simulink model "DriverInLoopGamingEngine"  (R2022b)
settings: Solver=ode3  StartTime=0.0  StopTime=inf  FixedStep=1e-3  RelTol=1e-3
StartFcn:
  | tg.load('DriverInLoopSpeedgoat');
  | tg.start;
StopFcn:
  | tg.stop;
model workspace (MAT data in the model file):
  DLCXref = [0 7.023 7.5 18 33 33.5 45 50 60]
  DLCYref = [0 0 -4.5 -4.25 -3.75 1.5 1.25 0 0]
  Downshift_Speeds = [9.5625  23.0625  36.5625  47.8125  59.0625  68.90625  78.75; 12.9375  26.4375  39.9375  51.1875  62.4375  72.84375  83.25; 16.3125  29.8125  43.3125  54.5625  65.8125  76.78125  87.75; 19.6875  33.1875  46.6875  57.9375  69.1875  80.71875  92.25]
  EngRevLim = 7000
  Pedal_Positions = [0.1 0.4 0.5 0.9]
  Upshift_Speeds = [12.9375  26.4375  39.9375  51.1875  62.4375  72.84375  83.25; 16.3125  29.8125  43.3125  54.5625  65.8125  76.78125  87.75; 19.6875  33.1875  46.6875  57.9375  69.1875  80.71875  92.25; 33  52.5  77.25  100.5  138.75  161.875  185]
  VEH.Mass = 1181
  VEH.StaticNormalFrontLoad.FR = 264.666666667
  VEH.StaticNormalFrontLoad.FL = 264.666666667
  VEH.StaticNormalRearLoad.RR = 322
  VEH.StaticNormalRearLoad.RL = 322
  VEH.WheelBase = 3.075
  VEH.FrontAxlePositionfromCG = 1.515
  VEH.RearAxlePositionfromCG = 1.504
  VEH.HeightCG = 0.134
  VEH.FrontalArea = 2.11
  VEH.DragCoefficient = 0.33
  VEH.NumberOfWheelsPerAxle = 2
  VEH.PitchMomentInertia = 1922.66666667
  VEH.RollMomentInertia = 432.333333333
  VEH.YawMomentInertia = 2066
  VEH.SteeringRatio = 18
  VEH.TrackWidth = 1.922
  VEH.SprungMass = 1096.72266667
  VEH.InitialLongPosition = -26
  VEH.InitialLatPosition = 76
  VEH.InitialVertPosition = 0
  VEH.InitialRollAngle = 0
  VEH.InitialPitchAngle = 0
  VEH.InitialYawAngle = -0.698131700798
  VEH.InitialLongVel = 0
  VEH.InitialLatVel = 0
  VEH.InitialVertVel = 0
  VEH.InitialRollRate = 0
  VEH.InitialPitchRate = 0
  VEH.InitialYawRate = 0
libraries: slrealtimeutilitieslib x3, slrealtimeiplib x3, sim3dlib x2, sim3dautolib x1, vrlib x1, simulink x1
settings Model: Creator=ashankar  LastModifiedBy=RASLab-Distributed
settings SolverCC: AlgebraicLoopSolver=TrustRegion  AutoInsertRateTranBlk=on  InsertRTBMode=Never (minimum delay)  DecoupledContinuousIntegration=on
settings DebuggingCC: UnconnectedInputMsg=warning  UnconnectedOutputMsg=warning  UnconnectedLineMsg=warning  SFMachineParentedDataDiag=warning  ArithmeticOperatorsInVariantConditions=warning
settings ModelReferenceCC: EnableRefExpFcnMdlSchedulingChecks=on
settings SFSimCC: SimUseLocalCustomCode=off  CustomCodeUndefinedFunction=UseInterfaceOnly
settings RTWCC: RTWUseLocalCustomCode=off  DLArmComputeVersion=19.05

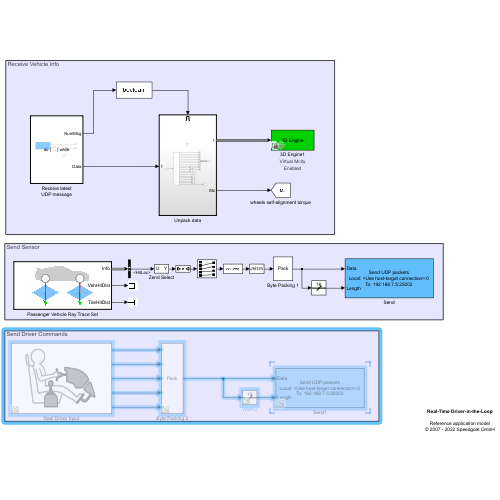
[thumbnail: Simulink's stored preview of the top-level diagram]
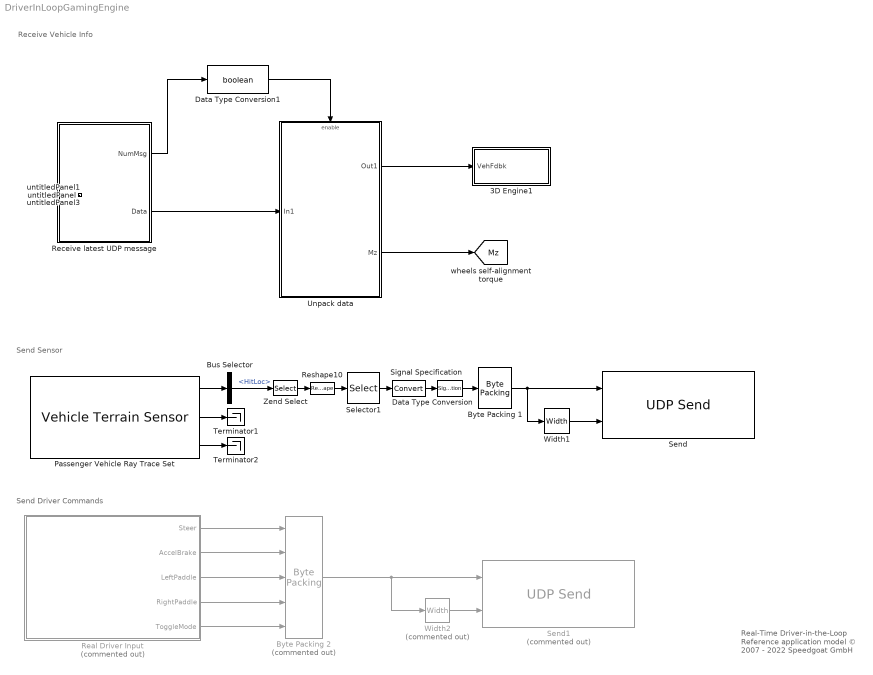
== system DriverInLoopGamingEngine ==
  note: Send Sensor
  note: Receive Vehicle Info
  note: Send Driver Commands
  note: Real-Time Driver-in-the-Loop
      |
      | Reference application model
      | © 2007 - 2022 Speedgoat GmbH
  3D Engine1 : Subsystem  Variant=on  VariantControlMode=label  LabelModeActiveChoice=1  mask(3D Engine){engine3D=Enabled, SceneDesc=Virtual Mcity, dt3D=0.02, defaultPos=Recommended for scene, X_o=-26.0, Y_o=76.0, Z_o=0.0, phi_o=0, theta_o=0, psi_o=-40*pi/180}
      mask prompts: engine3D "3D Engine"; SceneDesc "Scene:"; dt3D "Engine frame rate, dt3D [s]:"; X_o "Initial longitudinal position, X_o [m]:"; Y_o "Initial lateral position, Y_o [m]:"; Z_o "Initial vertical position, Z_o [m]:"; phi_o "Initial roll angle, phi_o [rad]:"; theta_o "Initial pitch angle, theta_o [rad]:"; psi_o "Initial yaw angle, psi_o [rad]:"
      mask help: This subsystem contains the interface blocks which permit the display of the vehicle in the 3D virtual environment. Enable it to view the simulation progress, disable it to inhibit the display.
      mask init:
      | switch get_param(gcb,'engine3D')
      |     case 'Disabled'
      |         set_param(gcb,'OverrideUsingVariant','0')
      |         try
      |             set_param([bdroot '/Environment/Ground Feedback'],'OverrideUsingVariant','0')
      |         catch
      |             disp('Warning: No ground feedback sensor not set')
      |         end
      |     case 'Enabled'
      |         set_param(gcb,'OverrideUsingVariant','1')
      |         try
      |             set_param([bdroot '/Environment/Ground Feedback'],'OverrideUsingVariant','1')
      |         catch
      |             disp('Warning: No ground feedback sensor not set')
      |         end
      |     otherwise
      |         set_param(gcb,'OverrideUsingVariant','0')
      | end
      settings: AttributesFormatString=|
      | %<SceneDesc>
      | %<engine3D>
      mask Help: eval('vdynblkshelp(''vdynblks3dengine'')');
      mask TypeOptions engine3D: Enabled | Disabled
      mask Callback engine3D:
      | switch get_param(gcb,'engine3D')
      |     case 'Disabled'
      |         set_param(gcb,'OverrideUsingVariant','0')
      |     case 'Enabled'
      |        set_param(gcb,'OverrideUsingVariant','1')
      |     otherwise
      |        set_param(gcb,'OverrideUsingVariant','0')
      | end
      mask TypeOptions SceneDesc: 3D Engine/Simulation 3D Scene Configuration/SceneDesc
      mask Callback SceneDesc:
      | defaultStatus = get_param(gcb,'defaultPos');
      | if strcmp(defaultStatus,'Recommended for scene')
      | sceneType = get_param(gcb,'SceneDesc');
      | switch sceneType
      |     case 'Straight road'
      |         set_param(gcb,'X_o', '-118')
      |         set_param(gcb,'Y_o', '3.125')
      |         set_param(gcb,'Z_o', '0')
      |         set_param(gcb,'phi_o', '0')
      |         set_param(gcb,'theta_o', '0')
      |         set_param(gcb,'psi_o', '0')
      |     case 'Curved road'
      |         set_param(gcb,'X_o', '0.2')
      |         set_param(gcb,'Y_o', '-1605.0')
      |         set_param(gcb,'Z_o', '0')
      |         set_param(gcb,'phi_o', '0')
      |         set_param(gcb,'theta_o', '0')
      |         set_param(gcb,'psi_o', '-156*pi/180')
      |     case 'Parking lot'
      |         set_param(gcb,'X_o', '-104.0')
      |         set_param(gcb,'Y_o', '-9.7')
      |         set_param(gcb,'Z_o', '0')
      |         set_param(gcb,'phi_o', '0')
      |         set_param(gcb,'theta_o', '0')
      |         set_param(gcb,'psi_o', '0')
      |     case 'Double lane change'
      |         set_param(gcb,'X_o', '0')
      |         set_param(gcb,'Y_o', '3.125')
      |         set_param(gcb,'Z_o', '0')
      |         set_param(gcb,'phi_o', '0')
      |         set_param(gcb,'theta_o', '0')
      |         set_param(gcb,'psi_o', '0')
      |     case 'Open surface'
      |         set_param(gcb,'X_o', '0')
      |         set_param(gcb,'Y_o', '0')
      |         set_param(gcb,'Z_o', '0')
      |         set_param(gcb,'phi_o', '0')
      |         set_param(gcb,'theta_o', '0')
      |         set_param(gcb,'psi_o', '0')
      |     case 'US highway'
      |         set_param(gcb,'X_o', '3592.00')
      |         set_param(gcb,'Y_o', '2617.00')
      |         set_param(gcb,'Z_o', '-1.0')
      |         set_param(gcb,'phi_o', '0')
      |         set_param(gcb,'theta_o', '0')
      |         set_param(gcb,'psi_o', '0')
      |     case 'US city block'
      |         set_param(gcb,'X_o', '-125.19')
      |         set_param(gcb,'Y_o', '1.65')
      |         set_param(gcb,'Z_o', '-0.04')
      |         set_param(gcb,'phi_o', '0')
      |         set_param(gcb,'theta_o', '0')
      |         set_param(gcb,'psi_o', '0')
      |     case 'Large parking lot'
      |         set_param(gcb,'X_o', '45.0')
      |         set_param(gcb,'Y_o', '54.7')
      |         set_param(gcb,'Z_o', '0.0')
      |         set_param(gcb,'phi_o', '0')
      |         set_param(gcb,'theta_o', '0')
      |         set_param(gcb,'psi_o', '-pi/2')
      |     case 'Virtual Mcity'
      |         set_param(gcb,'X_o', '-26.0')
      |         set_param(gcb,'Y_o', '76.0')
      |         set_param(gcb,'Z_o', '0.0')
      |         set_param(gcb,'phi_o', '0')
      |         set_param(gcb,'theta_o', '0')
      |         set_param(gcb,'psi_o', '-40*pi/180')
      |     otherwise
      |         set_param(gcb,'X_o', '0')
      |         set_param(gcb,'Y_o', '0')
      |         set_param(gcb,'Z_o', '0')
      |         set_param(gcb,'phi_o', '0')
      |         set_param(gcb,'theta_o', '0')
      |         set_param(gcb,'psi_o', '0')
      | end
      | end
      mask TypeOptions defaultPos: Recommended for scene | User-specified
      mask DialogControl engineConfig Prompt: 3D Engine Settings
      mask DialogControl posSetup Prompt: Initial vehicle position
      mask DialogControl posSetupDesc Prompt: To use these initial vehicle positions, first Apply the initial values and then click Update the model workspaces with the initial values.
      mask DialogControl setModelPos Prompt: Update model workspaces with initial values
      mask DialogControl setModelPos Callback:
      | if strcmp(get_param(bdroot(gcb),'SimulationStatus'),'stopped')
      |     sceneType = get_param(gcb,'SceneDesc');
      |     rootModel = bdroot(gcb);
      |     ws = get_param(rootModel, 'modelworkspace');
      |     VEH = getVariable(ws,'VEH');
      |     ParamList={'X_o',[1,1],{};'Y_o',[1,1],{};'Z_o',[1,1],{};'phi_o',[1,1],{'gte',-pi/2;'lte',pi/2};'theta_o',[1,1],{'gte',-pi/2;'lte',pi/2};'psi_o',[1,1],{'gte',-2*pi;'lte',2*pi}};
      |     paramStruct = autoblkscheckparams(gcb, '3D Engine',ParamList);
      |     VEH.InitialLongPosition = paramStruct.X_o;
      |     VEH.InitialLatPosition = paramStruct.Y_o;
      |     VEH.InitialVertPosition = paramStruct.Z_o;
      |     VEH.InitialRollAngle = paramStruct.phi_o;
      |     VEH.InitialPitchAngle = paramStruct.theta_o;
      |     VEH.InitialYawAngle = paramStruct.psi_o;
      |     assignin(ws,'VEH',VEH);
      |     modelList = {'PassVeh14DOF','PassVeh7DOF'};
      |     for idx =1:length(modelList)
      | %         try
      |             load_system(modelList{idx});
      |             ws = get_param(modelList{idx}, 'modelworkspace');
      |             assignin(ws,'VEH',VEH);
      |             save_system(modelList{idx});
      |             close_system(modelList{idx});
      | %         catch
      | %             disp(['Cannot find ' modelList{idx}])
      | %         end
      |     end
      | end
      mask Display: disp('3D Engine')
  Bus Selector : BusSelector  OutputSignals=HitLoc
  Byte Packing 1 : slrealtimeutilitieslib/Byte Packing  MaskPackedDataType=uint8  MaskUnpackedDataTypes={['single']}  MaskAlignment=1
  Byte Packing 2 : slrealtimeutilitieslib/Byte Packing  Commented=on  MaskPackedDataType=uint8  MaskUnpackedDataTypes={'double','double','boolean','boolean','boolean'}  MaskAlignment=1
  Data Type Conversion : DataTypeConversion  SaturateOnIntegerOverflow=off  RndMeth=Floor
  Data Type Conversion1 : DataTypeConversion  OutDataTypeStr=boolean  SaturateOnIntegerOverflow=off  RndMeth=Floor
  Passenger Vehicle Ray Trace Set : sim3dlib/Vehicle Terrain Sensor  Priority=1  ActorTag=SimulinkVehicle1  VehExtEn=Constant  TireRadiiExt=Constant  VehCntrLngthVal=0  TireRadiiVal=0  VehRayLngth=10  LfRayLngth=20  RfRayLngth=20  LrRayLngth=20  RrRayLngth=20  VehRayOffset=0  LfRayOffset=-1  RfRayOffset=-1  LrRayOffset=-1  RrRayOffset=-1  VehEn=on  LfEn=on  RfEn=on  LrEn=on  RrEn=on  DbgEn=off  Ts=-1  aMode=aMode
  Real Driver Input : Subsystem  Commented=on
      mask Display: image('LongitudinalDriver.png'); % Use "Edit Image" on toolstrip to change.
  Receive latest UDP message : Subsystem  TreatAsAtomicUnit=on
  Reshape10 : Reshape  OutputDimensionality=Row vector (2-D)
  Selector1 : Selector  InputPortWidth=5  IndexOptions=Index vector (dialog)  Indices=[2:5]  OutputSizes=1
  Send : slrealtimeiplib/UDP Send  useHostTargetConn=on  toAddress=target_ip  toPort=25002  sampleTime=-1  enableMessage=off  ipAddress=172.16.19.29  localPort=-1
  Send1 : slrealtimeiplib/UDP Send  Commented=on  useHostTargetConn=on  toAddress=target_ip  toPort=25003  sampleTime=-1  enableMessage=off  ipAddress=172.16.19.29  localPort=-1
  Signal Specification : SignalSpecification  Unit=m
  Terminator1 : Terminator
  Terminator2 : Terminator
  Unpack data : Subsystem
  Width1 : Width
  Width2 : Width  Commented=on
  Zend Select : Selector  NumberOfDimensions=2  InputPortWidth=3  IndexOptions=Select all,Index vector (dialog)  Indices=[1 3],3  OutputSizes=1,1
  untitledPanel : Subsystem  Tag=HiddenForWebPanel  IsWebBlockPanel=on
  untitledPanel1 : Subsystem  Tag=HiddenForWebPanel  IsWebBlockPanel=on
  untitledPanel3 : Subsystem  Tag=HiddenForWebPanel  IsWebBlockPanel=on
  tag scope: Mz=global
  wires:
  Reshape10/1 -> Selector1/1
  Bus Selector/1 -> Zend Select/1  "<HitLoc>"
  Zend Select/1 -> Reshape10/1
  Passenger Vehicle Ray Trace Set/3 -> Terminator2/1
  Passenger Vehicle Ray Trace Set/1 -> Bus Selector/1
  Width1/1 -> Send/2
  Passenger Vehicle Ray Trace Set/2 -> Terminator1/1
  Byte Packing 1/1 -> Width1/1, Send/1
  Width2/1 -> Send1/2
  Byte Packing 2/1 -> Width2/1, Send1/1
  Real Driver Input/2(AccelBrake) -> Byte Packing 2/2
  Real Driver Input/3(LeftPaddle) -> Byte Packing 2/3
  Real Driver Input/1(Steer) -> Byte Packing 2/1
  Real Driver Input/4(RightPaddle) -> Byte Packing 2/4
  Selector1/1 -> Data Type Conversion/1
  Data Type Conversion/1 -> Signal Specification/1
  Signal Specification/1 -> Byte Packing 1/1
  Data Type Conversion1/1 -> Unpack data/Enable
  Receive latest UDP message/2(Data) -> Unpack data/1(In1)
  Receive latest UDP message/1(NumMsg) -> Data Type Conversion1/1
  Real Driver Input/5(ToggleMode) -> Byte Packing 2/5
  Unpack data/2(Mz) -> [Mz]
  Unpack data/1(Out1) -> 3D Engine1/1(VehFdbk)

== system DriverInLoopGamingEngine/3D Engine1 ==
  note: 1) Add Subsystem or Model blocks as valid variant choices.
      | 2) You cannot connect blocks at this level. At simulation, connectivity is automatically
      | determined, based on the active variant and port name matching.
  VehFdbk : Inport
  3D Engine : Subsystem  VariantControl=1
  3D Engine Disabled : Subsystem  VariantControl=0

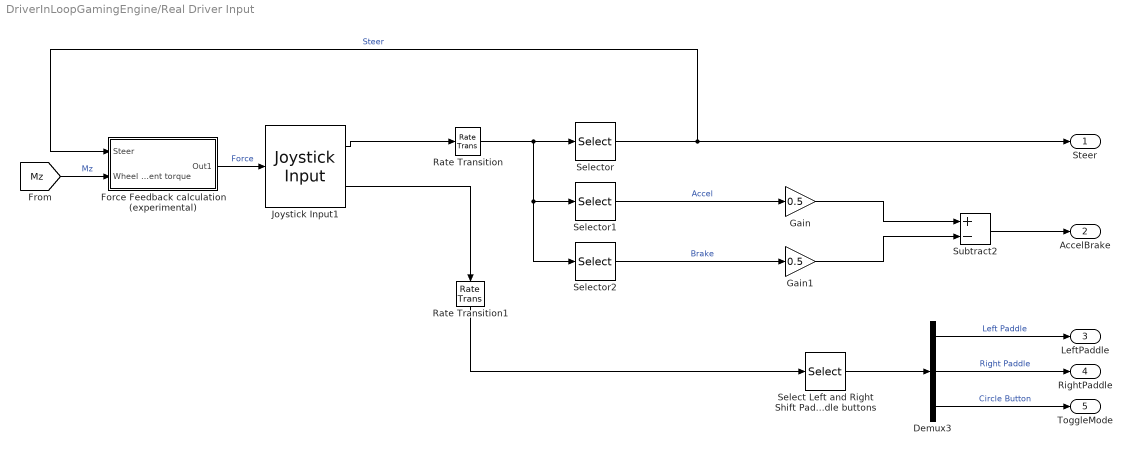
== system DriverInLoopGamingEngine/Real Driver Input ==
  Demux3 : Demux  Outputs=3
  Force Feedback calculation (experimental) : Subsystem
  Gain : Gain  Gain=0.5
  Gain1 : Gain  Gain=0.5
  Joystick Input1 : vrlib/Joystick Input  joyid=1  adjustports=on  forcefeed=on
  Rate Transition : RateTransition  Deterministic=off
  Rate Transition1 : RateTransition  Deterministic=off
  Select Left and Right Shift Paddle buttons : Selector  InputPortWidth=25  IndexOptions=Index vector (dialog)  Indices=[6 5 3]  OutputSizes=1
  Selector : Selector  InputPortWidth=4  IndexOptions=Index vector (dialog)  Indices=1  OutputSizes=1
  Selector1 : Selector  InputPortWidth=4  IndexOptions=Index vector (dialog)  Indices=2  OutputSizes=1
  Selector2 : Selector  InputPortWidth=4  IndexOptions=Index vector (dialog)  Indices=3  OutputSizes=1
  Subtract2 : Sum  Inputs=+-
  Steer : Outport  VectorParamsAs1DForOutWhenUnconnected=off
  AccelBrake : Outport  Port=2  VectorParamsAs1DForOutWhenUnconnected=off
  LeftPaddle : Outport  Port=3  VectorParamsAs1DForOutWhenUnconnected=off
  RightPaddle : Outport  Port=4  VectorParamsAs1DForOutWhenUnconnected=off
  ToggleMode : Outport  Port=5  VectorParamsAs1DForOutWhenUnconnected=off
  wires:
  Joystick Input1/1 -> Rate Transition/1
  Rate Transition1/1 -> Select Left and Right Shift Paddle buttons/1
  Demux3/2 -> RightPaddle/1  "Right Paddle"
  Demux3/1 -> LeftPaddle/1  "Left Paddle"
  Select Left and Right Shift Paddle buttons/1 -> Demux3/1
  Rate Transition/1 -> Selector2/1, Selector1/1, Selector/1
  Joystick Input1/2 -> Rate Transition1/1
  Selector1/1 -> Gain/1  "Accel"
  Selector2/1 -> Gain1/1  "Brake"
  Gain/1 -> Subtract2/1
  Gain1/1 -> Subtract2/2
  Subtract2/1 -> AccelBrake/1
  Demux3/3 -> ToggleMode/1  "Circle Button"
  Selector/1 -> Steer/1, Force Feedback calculation (experimental)/1(Steer)  "Steer"
  [Mz] -> Force Feedback calculation (experimental)/2(Wheel alignment torque)  "Mz"
  Force Feedback calculation (experimental)/1(Out1) -> Joystick Input1/1  "Force"

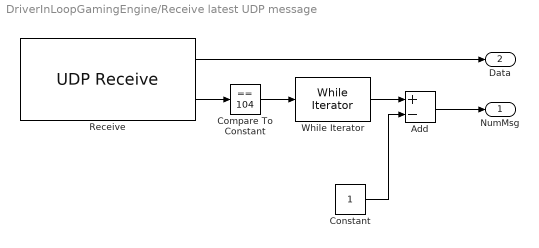
== system DriverInLoopGamingEngine/Receive latest UDP message ==
  Add : Sum  Inputs=+-
  Compare To Constant : simulink/Logic and Bit Operations/Compare To Constant  relop===  const=104  OutDataTypeStr=boolean
  Constant : Constant  OutDataTypeStr=Inherit: Inherit via back propagation  SampleTime=-1
  Receive : slrealtimeiplib/UDP Receive  useHostTargetConn=on  ipAddress=host_ip  localPort=25001  rcvWidth=104  rcvFmAny=off  fmAddress=target_ip  sampleTime=-1  enableMessage=off  maxPackets=1
  While Iterator : WhileIterator  MaxIters=10  WhileBlockType=do-while  ShowIterationPort=on
  NumMsg : Outport
  Data : Outport  Port=2
  wires:
  Receive/2 -> Compare To Constant/1
  Compare To Constant/1 -> While Iterator/1
  While Iterator/1 -> Add/1
  Constant/1 -> Add/2
  Receive/1 -> Data/1
  Add/1 -> NumMsg/1

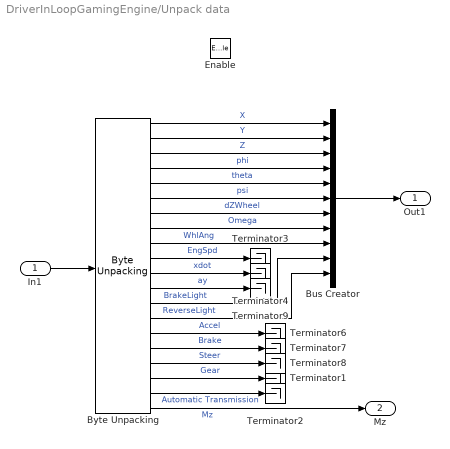
== system DriverInLoopGamingEngine/Unpack data ==
  In1 : Inport
  Enable : EnablePort
  Bus Creator : BusCreator  Inputs=11
  "Byte Unpacking " : slrealtimeutilitieslib/Byte Unpacking  MaskUnpackedDataTypes={'single','single','single','single','single','single','single','single','single','single','single','single','boolean','boolean','single','single','single','int8','int8','single'}  MaskUnpackedDataSizes={[1],[1],[1],[1],[1],[1],[4],[4],[4],[1],[1],[1],[1],[1],[1],[1],[1],[1],[1],[1]}  MaskAlignment=1
  Terminator{1..4,6..9} (8 alike) : Terminator
  Out1 : Outport
  Mz : Outport  Port=2
  wires:
  "Byte Unpacking "/8 -> Bus Creator/8  "Omega"
  "Byte Unpacking "/16 -> Terminator7/1  "Brake"
  "Byte Unpacking "/7 -> Bus Creator/7  "dZWheel"
  "Byte Unpacking "/4 -> Bus Creator/4  "phi"
  "Byte Unpacking "/17 -> Terminator8/1  "Steer"
  "Byte Unpacking "/9 -> Bus Creator/9  "WhlAng"
  "Byte Unpacking "/15 -> Terminator6/1  "Accel"
  "Byte Unpacking "/2 -> Bus Creator/2  "Y"
  "Byte Unpacking "/10 -> Terminator3/1  "EngSpd"
  In1/1 -> "Byte Unpacking "/1
  "Byte Unpacking "/3 -> Bus Creator/3  "Z"
  "Byte Unpacking "/14 -> Bus Creator/11  "ReverseLight"
  "Byte Unpacking "/11 -> Terminator4/1  "xdot"
  "Byte Unpacking "/1 -> Bus Creator/1  "X"
  "Byte Unpacking "/6 -> Bus Creator/6  "psi"
  "Byte Unpacking "/5 -> Bus Creator/5  "theta"
  Bus Creator/1 -> Out1/1
  "Byte Unpacking "/18 -> Terminator1/1  "Gear"
  "Byte Unpacking "/19 -> Terminator2/1  "Automatic Transmission"
  "Byte Unpacking "/20 -> Mz/1  "Mz"
  "Byte Unpacking "/12 -> Terminator9/1  "ay"
  "Byte Unpacking "/13 -> Bus Creator/10  "BrakeLight"

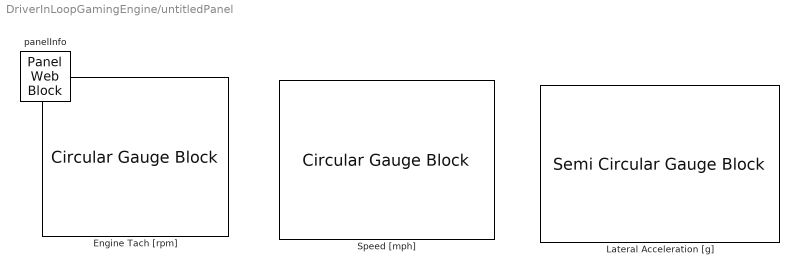
== system DriverInLoopGamingEngine/untitledPanel ==
  Engine Tach [rpm] : CircularGaugeBlock  Tag=HiddenForWebPanel  PanelInfo="{\"height\":159,\"left\":37,\"panelId\":\"panelId-ef65929c-f6fa-498a-ac85-12dbb8e733e6\",\"top\":41,\"type\":\"panelChild\",\"version\":\"2019b\",\"width\":186,\"zIndex\":1500002}"  ScaleMax=8000  TickInterval=1000
  Lateral Acceleration [g] : SemiCircularGaugeBlock  Tag=HiddenForWebPanel  PanelInfo="{\"height\":157,\"left\":535,\"panelId\":\"panelId-ef65929c-f6fa-498a-ac85-12dbb8e733e6\",\"top\":49,\"type\":\"panelChild\",\"version\":\"2019b\",\"width\":239,\"zIndex\":1500004}"  ScaleMin=-1  ScaleMax=1  TickInterval=0.5
  Speed [mph] : CircularGaugeBlock  Tag=HiddenForWebPanel  PanelInfo="{\"height\":159,\"left\":274,\"panelId\":\"panelId-ef65929c-f6fa-498a-ac85-12dbb8e733e6\",\"top\":44,\"type\":\"panelChild\",\"version\":\"2019b\",\"width\":215,\"zIndex\":1500006}"
  panelInfo : PanelWebBlock  Tag=HiddenForWebPanel  PanelInfo="{\"compacted\":false,\"height\":242,\"isActiveTab\":true,\"labels\":{\"label3773900240\":{\"left\":\"361\",\"settings\":{\"backgroundColor\":\"rgba(0, 0, 0, 0)\",\"bold\":false,\"font\":\"Arial\",\"fontColor\":\"black\",\"fontSize\":0.65,\"italicized\":false,\"underlined\":false},\"text\":\"Velocity\",\"top\":\"210\"},\"label4823130022\":{\"left\":\"606\",\"settings\":{\"backgroundColor\":\"rgba(0, 0, 0, 0)\",\"bold\":false,\"font\":\"Arial\",\"fontColor\":\"black\",\"fontSize\":0.65,\"italicized\":false,\"underlined\":false},\"text\":\"Lateral Acceleration\",\"top\":\"212\"},\"label7777085124\":{\"left\":\"98\",\"settings\":{\"backgroundColor\":\"rgba(0, 0, 0, 0)\",\"bold\":false,\"font\":\"Arial\",\"fontColor\":\"black\",\"fontSize\":0.65,\"italicized\":false,\"underlined\":false},\"text\":\"Engine RPM\",\"top\":\"209\"},\"label9552319808\":{\"left\":\"17\",\"settings\":{\"backgroundColor\":\"rgba(0, 0, 0, 0)\",\"bold\":false,\"font\":\"Arial\",\"fontColor\":\"black\",\"fontSize\":0.88,\"italicized\":false,\"underlined\":false},\"text\":\"Vehicle Response\",\"top\":\"10\"}},\"left\":1003,\"name\":\"untitledPanel\",\"panelId\":\"panelId-ef65929c-f6fa-498a-ac85-12dbb8e733e6\",\"tabIndex\":0,\"tabbedSetId\":\"tabbedSet0208619071\",\"top\":312,\"type\":\"panel\",\"version\":\"2019b\",\"visible\":true,\"width\":823,\"zIndex\":1500002}"  PanelSnapshot=<binary blob, 64776 chars, not shown>

== system DriverInLoopGamingEngine/untitledPanel1 ==
  Gear : LinearGaugeBlock  Tag=HiddenForWebPanel  PanelInfo="{\"height\":68,\"left\":11,\"panelId\":\"panelId-ef8ee8f9-362c-40cc-b79e-7f67918ef485\",\"top\":156,\"type\":\"panelChild\",\"version\":\"2019b\",\"width\":172,\"zIndex\":1500002}"  ScaleMin=-1  ScaleMax=5  TickInterval=1
  Lamp : LampBlock  Tag=HiddenForWebPanel  PanelInfo="{\"height\":82,\"left\":54,\"panelId\":\"panelId-ef8ee8f9-362c-40cc-b79e-7f67918ef485\",\"top\":37,\"type\":\"panelChild\",\"version\":\"2019b\",\"width\":90,\"zIndex\":1500004}"
  panelInfo : PanelWebBlock  Tag=HiddenForWebPanel  PanelInfo="{\"compacted\":false,\"height\":248,\"isActiveTab\":true,\"labels\":{\"label1969274100\":{\"left\":\"16\",\"settings\":{\"backgroundColor\":\"rgba(0, 0, 0, 0)\",\"bold\":false,\"font\":\"Arial\",\"fontColor\":\"black\",\"fontSize\":0.81,\"italicized\":false,\"underlined\":false},\"text\":\"Transmission\",\"top\":\"10\"},\"label7939780652\":{\"left\":\"75\",\"settings\":{\"backgroundColor\":\"rgba(0, 0, 0, 0)\",\"bold\":false,\"font\":\"Arial\",\"fontColor\":\"black\",\"fontSize\":0.61,\"italicized\":false,\"underlined\":false},\"text\":\"Auto On\\/Off\",\"top\":\"124\"},\"label9948480676\":{\"left\":\"89\",\"settings\":{\"backgroundColor\":\"rgba(0, 0, 0, 0)\",\"bold\":false,\"font\":\"Arial\",\"fontColor\":\"black\",\"fontSize\":0.61,\"italicized\":false,\"underlined\":false},\"text\":\"Gear\",\"top\":\"227\"}},\"left\":1641,\"name\":\"untitledPanel1\",\"panelId\":\"panelId-ef8ee8f9-362c-40cc-b79e-7f67918ef485\",\"tabIndex\":0,\"tabbedSetId\":\"tabbedSet0851869161\",\"top\":44,\"type\":\"panel\",\"version\":\"2019b\",\"visible\":true,\"width\":192,\"zIndex\":1500004}"  PanelSnapshot=<binary blob, 14408 chars, not shown>

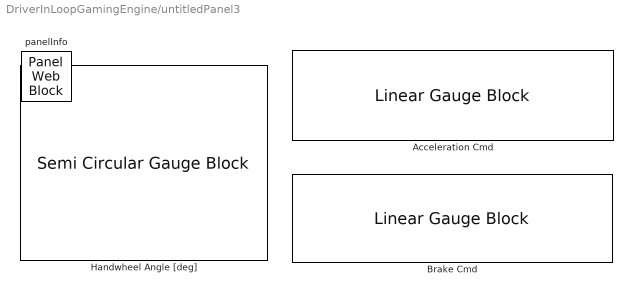
== system DriverInLoopGamingEngine/untitledPanel3 ==
  Acceleration Cmd : LinearGaugeBlock  Tag=HiddenForWebPanel  PanelInfo="{\"height\":90,\"left\":286,\"panelId\":\"panelId-d807b6de-8dbd-4274-bd39-1005cdfde51f\",\"top\":14,\"type\":\"panelChild\",\"version\":\"2019b\",\"width\":321,\"zIndex\":1500004}"  ScaleMax=1
  Brake Cmd : LinearGaugeBlock  Tag=HiddenForWebPanel  PanelInfo="{\"height\":88,\"left\":286,\"panelId\":\"panelId-d807b6de-8dbd-4274-bd39-1005cdfde51f\",\"top\":138,\"type\":\"panelChild\",\"version\":\"2019b\",\"width\":320,\"zIndex\":1500006}"  ScaleMax=1
  Handwheel Angle [deg] : SemiCircularGaugeBlock  Tag=HiddenForWebPanel  PanelInfo="{\"height\":195,\"left\":14,\"panelId\":\"panelId-d807b6de-8dbd-4274-bd39-1005cdfde51f\",\"top\":29,\"type\":\"panelChild\",\"version\":\"2019b\",\"width\":247,\"zIndex\":1500002}"  ScaleMin=-450  ScaleMax=450  TickInterval=90
  panelInfo : PanelWebBlock  Tag=HiddenForWebPanel  PanelInfo="{\"compacted\":false,\"height\":247,\"isActiveTab\":true,\"labels\":{\"label11269868162\":{\"left\":\"14\",\"settings\":{\"backgroundColor\":\"rgba(0, 0, 0, 0)\",\"bold\":false,\"font\":\"Arial\",\"fontColor\":\"black\",\"fontSize\":0.79,\"italicized\":false,\"underlined\":false},\"text\":\"Driver Input\",\"top\":\"9\"},\"label18147236863\":{\"left\":\"397\",\"settings\":{\"backgroundColor\":\"rgba(0, 0, 0, 0)\",\"bold\":false,\"font\":\"Arial\",\"fontColor\":\"black\",\"fontSize\":0.6,\"italicized\":false,\"underlined\":false},\"text\":\"Acceleration Command\",\"top\":\"108\"},\"label19057919370\":{\"left\":\"88\",\"settings\":{\"backgroundColor\":\"rgba(0, 0, 0, 0)\",\"bold\":false,\"font\":\"Arial\",\"fontColor\":\"black\",\"fontSize\":0.6,\"italicized\":false,\"underlined\":false},\"text\":\"Steering Wheel Angle\",\"top\":\"202\"},\"label19133758561\":{\"left\":\"408\",\"settings\":{\"backgroundColor\":\"rgba(0, 0, 0, 0)\",\"bold\":false,\"font\":\"Arial\",\"fontColor\":\"black\",\"fontSize\":0.6,\"italicized\":false,\"underlined\":false},\"text\":\"Brake Command\",\"top\":\"230\"}},\"left\":996,\"name\":\"untitledPanel3\",\"panelId\":\"panelId-d807b6de-8dbd-4274-bd39-1005cdfde51f\",\"tabIndex\":0,\"tabbedSetId\":\"tabbedSet5234037390\",\"top\":44,\"type\":\"panel\",\"version\":\"2019b\",\"visible\":true,\"width\":619,\"zIndex\":1500008}"  PanelSnapshot=<binary blob, 45480 chars, not shown>

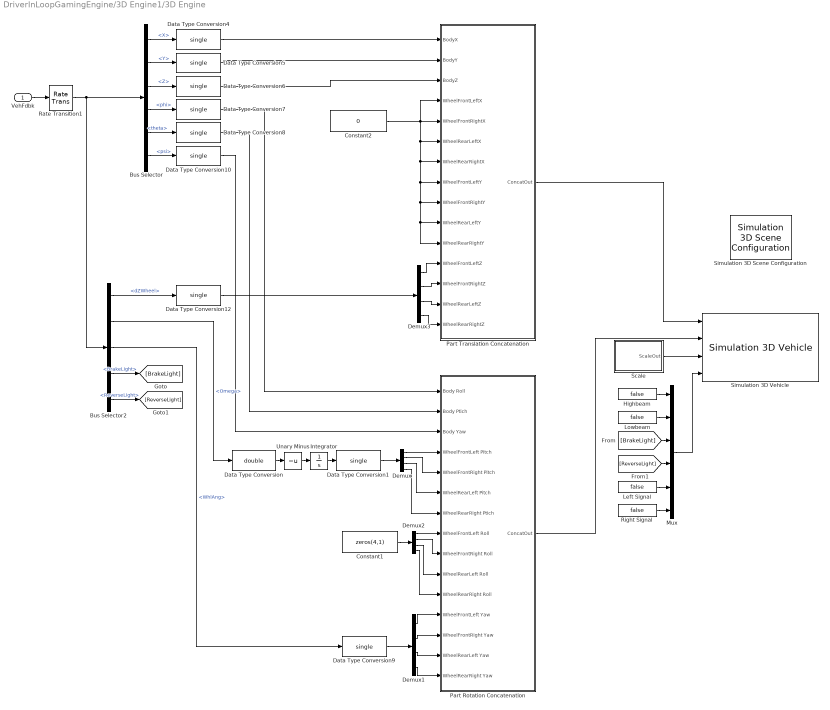
== system DriverInLoopGamingEngine/3D Engine1/3D Engine ==
  VehFdbk : Inport
  Bus Selector : BusSelector  OutputSignals=X,Y,Z,phi,theta,psi
  Bus Selector2 : BusSelector  OutputSignals=dZWheel,Omega,WhlAng,BrakeLight,ReverseLight
  Constant1 : Constant  Value=zeros(4,1)  OutDataTypeStr=single
  Constant2 : Constant  Value=0  OutDataTypeStr=single
  Data Type Conversion : DataTypeConversion  OutDataTypeStr=double  SaturateOnIntegerOverflow=off  RndMeth=Floor
  Data Type Conversion{1,4..10,12} (9 alike) : DataTypeConversion  OutDataTypeStr=single  SaturateOnIntegerOverflow=off  RndMeth=Floor
  Demux{,1..3} (4 alike) : Demux
  Highbeam : Constant  Value=false
  Integrator : Integrator  WrapState=on  WrappedStateUpperValue=2*pi  WrappedStateLowerValue=0  ZeroCross=off
  Left Signal : Constant  Value=false
  Lowbeam : Constant  Value=false
  Mux : Mux  Inputs=6
  Part Rotation Concatenation : Subsystem
  Part Translation Concatenation : Subsystem
  Rate Transition1 : RateTransition  OutPortSampleTime=dt3D
  Right Signal : Constant  Value=false
  Scale : Subsystem
  Simulation 3D Scene Configuration : sim3dlib/Simulation 3D Scene Configuration  Priority=0  ProjectFormat=Default Scenes  SceneDesc=Virtual Mcity  ProjectName=C:\Program Files\MATLAB\R2022b\toolbox\shared\sim3d_projects\automotive_project\UE4\WindowsNoEditor\VehicleSimulation.exe  ScenePath=/Game/Maps/HwStrght  EnableOpenDRIVE=off  vehTagList={'Scene Origin';'SimulinkVehicle1'}  vehTag=SimulinkVehicle1  OpVisEn=off  Ts=dt3D  EnableWindow=on  EnableRemoteAccess=off  EnableWeather=off  SunAltitude=40.0  SunAzimuth=90  clouds=10  wind=1  fog=0  rain=0  EnableGeospatial=off  OriginHeight=200  OriginLatitude=40.744652  OriginLongitude=-73.988864  MapStyle=Aerial  AdditionalAssetIDs=[]  UseAdvancedSunSky=off  SolarTime=11  TimeZone=-5  Day=21  Month=9  Year=2022  UseDaylightSavingTime=on  DSTStartDay=10  DSTStartMonth=3  DSTEndDay=3  DSTEndMonth=11  DSTSwitchHour=2  sensorTag=MainCamera2  sensorId=2  sensorName=MainCamera2  mountLoc=Origin  offsetFlag=off  tmountOffset=[0, 0, 0]  rmountOffset=[0, 0, 0]  HorizontalResolution=1280  VerticalResolution=720  HorizontalFOV=60  mountPoint=[0 0 0]  mountOrientation=[0 0 0]  aMode=aMode  ID=2  GeoTrigger=Inactive
  Simulation 3D Vehicle : sim3dautolib/Simulation 3D Vehicle  Priority=-1  PassVehMesh=Muscle car  MeshPath=/MathWorksSimulation/Vehicles/Muscle/Meshes/SK_MuscleCar.SK_MuscleCar  VehColor=Red  ActorName=SimulinkVehicle1  VehLightsControl=on  HeadlightColor=[ 1, 1, 1 ]  HighBeamIntensity=100000  LowBeamIntensity=60000  HighBeamConeAngle=1.22  LowBeamConeAngle=1.22  LeftHeadlightOrientation=[ 0, 0 ]  RightHeadlightOrientation=[ 0, 0 ]  BrakelightIntensity=500  ReverselightIntensity=500  SignallightIntensity=500  SignallightPeriod=1  SignalPulseWidth=50  Translation=[VEH.InitialLongPosition VEH.InitialLatPosition -VEH.InitialVertPosition; 0 0 0; 0 0 0; 0 0 0; 0 0 0]  Rotation=[VEH.InitialRollAngle VEH.InitialPitchAngle VEH.InitialYawAngle; 0 0 0; 0 0 0; 0 0 0; 0 0 0]  Scale=ones( 5, 3 )  SampleTime=dt3D  ActorType=SimulinkVehicle  ID=1  aMode=2  ActorTag=SimulinkVehicle1
  Unary Minus : UnaryMinus
  wires:
  Unary Minus/1 -> Integrator/1
  Bus Selector2/1 -> Data Type Conversion12/1  "<dZWheel>"
  Rate Transition1/1 -> Bus Selector/1, Bus Selector2/1
  Scale/1(ScaleOut) -> Simulation 3D Vehicle/3
  Demux/4 -> Part Rotation Concatenation/7(WheelRearRight Ptich)
  Demux/3 -> Part Rotation Concatenation/6(WheelRearLeft Pitch)
  Demux/2 -> Part Rotation Concatenation/5(WheelFrontRight Pitch)
  Demux/1 -> Part Rotation Concatenation/4(WheelFrontLeft Pitch)
  Constant1/1 -> Demux2/1
  Bus Selector/4 -> Data Type Conversion7/1  "<phi>"
  Part Rotation Concatenation/1(ConcatOut) -> Simulation 3D Vehicle/2
  Part Translation Concatenation/1(ConcatOut) -> Simulation 3D Vehicle/1
  Data Type Conversion12/1 -> Demux3/1
  Demux3/4 -> Part Translation Concatenation/15(WheelRearRightZ)
  Demux3/3 -> Part Translation Concatenation/14(WheelRearLeftZ)
  Demux3/1 -> Part Translation Concatenation/12(WheelFrontLeftZ)
  Demux3/2 -> Part Translation Concatenation/13(WheelFrontRightZ)
  VehFdbk/1 -> Rate Transition1/1
  Data Type Conversion6/1 -> Part Translation Concatenation/3(BodyZ)
  Demux1/4 -> Part Rotation Concatenation/15(WheelRearRight Yaw)
  Demux1/3 -> Part Rotation Concatenation/14(WheelRearLeft Yaw)
  Demux2/1 -> Part Rotation Concatenation/8(WheelFrontLeft Roll)
  Demux2/2 -> Part Rotation Concatenation/9(WheelFrontRight Roll)
  Demux2/3 -> Part Rotation Concatenation/10(WheelRearLeft Roll)
  Demux2/4 -> Part Rotation Concatenation/11(WheelRearRight Roll)
  Bus Selector2/3 -> Data Type Conversion9/1  "<WhlAng>"
  Bus Selector2/2 -> Data Type Conversion/1  "<Omega>"
  Data Type Conversion9/1 -> Demux1/1
  Demux1/1 -> Part Rotation Concatenation/12(WheelFrontLeft Yaw)
  Demux1/2 -> Part Rotation Concatenation/13(WheelFrontRight Yaw)
  Integrator/1 -> Data Type Conversion1/1
  Data Type Conversion1/1 -> Demux/1
  Data Type Conversion8/1 -> Part Rotation Concatenation/2(Body Ptich)
  Data Type Conversion5/1 -> Part Translation Concatenation/2(BodyY)
  Data Type Conversion10/1 -> Part Rotation Concatenation/3(Body Yaw)
  Constant2/1 -> Part Translation Concatenation/5(WheelFrontRightX), Part Translation Concatenation/6(WheelRearLeftX), Part Translation Concatenation/7(WheelRearRightX), Part Translation Concatenation/8(WheelFrontLeftY), Part Translation Concatenation/9(WheelFrontRightY), Part Translation Concatenation/10(WheelRearLeftY), Part Translation Concatenation/11(WheelRearRightY), Part Translation Concatenation/4(WheelFrontLeftX)
  Data Type Conversion4/1 -> Part Translation Concatenation/1(BodyX)
  Data Type Conversion7/1 -> Part Rotation Concatenation/1(Body Roll)
  Bus Selector/1 -> Data Type Conversion4/1  "<X>"
  Bus Selector/2 -> Data Type Conversion5/1  "<Y>"
  Bus Selector/3 -> Data Type Conversion6/1  "<Z>"
  Bus Selector/5 -> Data Type Conversion8/1  "<theta>"
  Bus Selector/6 -> Data Type Conversion10/1  "<psi>"
  [BrakeLight] -> Mux/3
  Left Signal/1 -> Mux/5
  Right Signal/1 -> Mux/6
  Lowbeam/1 -> Mux/2
  [ReverseLight] -> Mux/4
  Mux/1 -> Simulation 3D Vehicle/4
  Highbeam/1 -> Mux/1
  Bus Selector2/4 -> [BrakeLight]  "<BrakeLight>"
  Bus Selector2/5 -> [ReverseLight]  "<ReverseLight>"
  Data Type Conversion/1 -> Unary Minus/1

== system DriverInLoopGamingEngine/3D Engine1/3D Engine Disabled ==
  VehFdbk : Inport
  Terminator : Terminator
  wires:
  VehFdbk/1 -> Terminator/1

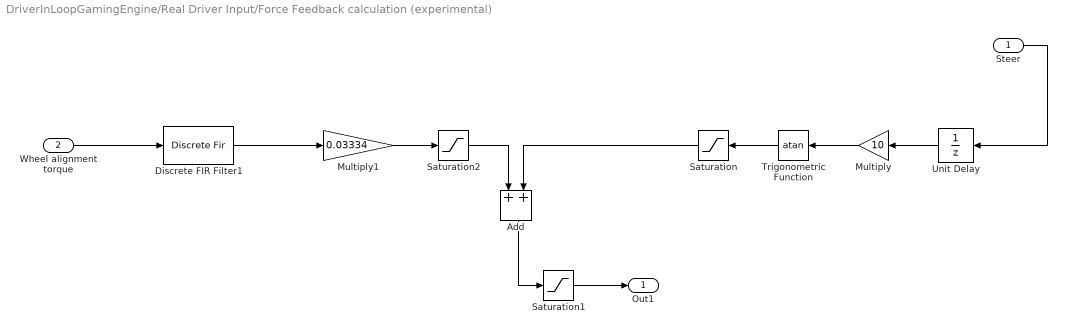
== system DriverInLoopGamingEngine/Real Driver Input/Force Feedback calculation (experimental) ==
  Steer : Inport
  Wheel alignment torque : Inport  Port=2
  Add : Sum
  Discrete FIR Filter1 : DiscreteFir  Coefficients=[0.1 0.1 0.1 0.1 0.1 0.1 0.1 0.1 0.1 0.1]
  Multiply : Gain  Gain=10
  Multiply1 : Gain  Gain=0.03334
  Saturation : Saturate  UpperLimit=0.6  LowerLimit=-0.6
  Saturation1 : Saturate  UpperLimit=1  LowerLimit=-1
  Saturation2 : Saturate  UpperLimit=0.6  LowerLimit=-0.6
  Trigonometric Function : Trigonometry  Operator=atan  OutputSignalType=real
  Unit Delay : UnitDelay  SampleTime=-1  HasFrameUpgradeWarning=on
  Out1 : Outport
  wires:
  Multiply/1 -> Trigonometric Function/1
  Unit Delay/1 -> Multiply/1
  Saturation1/1 -> Out1/1
  Saturation/1 -> Add/2
  Multiply1/1 -> Saturation2/1
  Trigonometric Function/1 -> Saturation/1
  Add/1 -> Saturation1/1
  Discrete FIR Filter1/1 -> Multiply1/1
  Saturation2/1 -> Add/1
  Steer/1 -> Unit Delay/1
  Wheel alignment torque/1 -> Discrete FIR Filter1/1

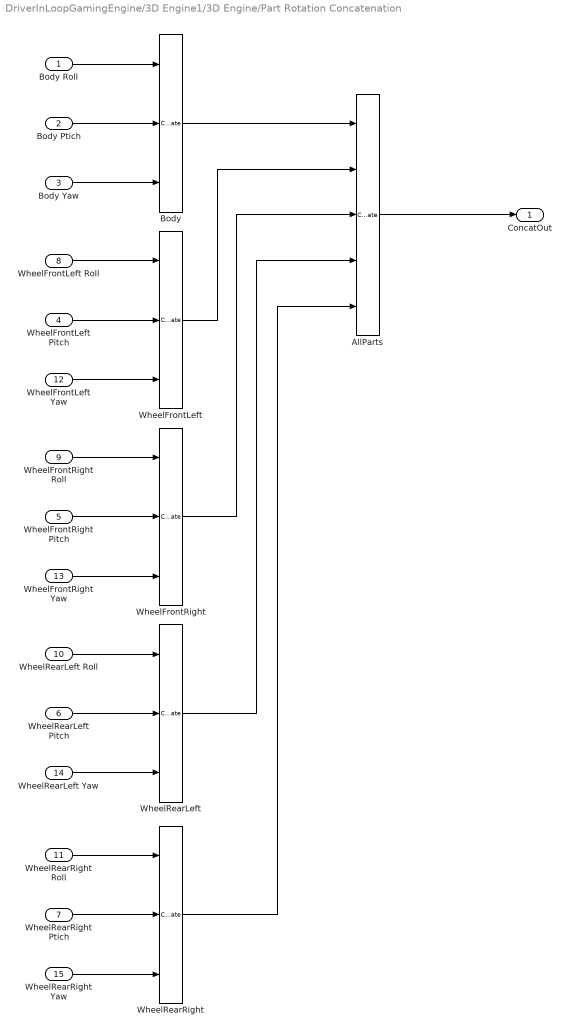
== system DriverInLoopGamingEngine/3D Engine1/3D Engine/Part Rotation Concatenation ==
  Body Roll : Inport
  Body Ptich : Inport  Port=2
  Body Yaw : Inport  Port=3
  WheelFrontLeft Pitch : Inport  Port=4
  WheelFrontRight Pitch : Inport  Port=5
  WheelRearLeft Pitch : Inport  Port=6
  WheelRearRight Ptich : Inport  Port=7
  WheelFrontLeft Roll : Inport  Port=8
  WheelFrontRight Roll : Inport  Port=9
  WheelRearLeft Roll : Inport  Port=10
  WheelRearRight Roll : Inport  Port=11
  WheelFrontLeft Yaw : Inport  Port=12
  WheelFrontRight Yaw : Inport  Port=13
  WheelRearLeft Yaw : Inport  Port=14
  WheelRearRight Yaw : Inport  Port=15
  AllParts : Concatenate  NumInputs=5  Mode=Multidimensional array
  Body : Concatenate  NumInputs=3  Mode=Multidimensional array  ConcatenateDimension=2
  WheelFrontLeft : Concatenate  NumInputs=3  Mode=Multidimensional array  ConcatenateDimension=2
  WheelFrontRight : Concatenate  NumInputs=3  Mode=Multidimensional array  ConcatenateDimension=2
  WheelRearLeft : Concatenate  NumInputs=3  Mode=Multidimensional array  ConcatenateDimension=2
  WheelRearRight : Concatenate  NumInputs=3  Mode=Multidimensional array  ConcatenateDimension=2
  ConcatOut : Outport  VectorParamsAs1DForOutWhenUnconnected=off
  wires:
  Body Yaw/1 -> Body/3
  WheelFrontLeft Yaw/1 -> WheelFrontLeft/3
  WheelFrontLeft/1 -> AllParts/2
  Body/1 -> AllParts/1
  WheelRearLeft/1 -> AllParts/4
  WheelFrontRight/1 -> AllParts/3
  WheelRearRight Yaw/1 -> WheelRearRight/3
  WheelRearLeft Yaw/1 -> WheelRearLeft/3
  AllParts/1 -> ConcatOut/1
  WheelRearRight/1 -> AllParts/5
  WheelFrontRight Yaw/1 -> WheelFrontRight/3
  Body Roll/1 -> Body/1
  Body Ptich/1 -> Body/2
  WheelFrontLeft Pitch/1 -> WheelFrontLeft/2
  WheelFrontLeft Roll/1 -> WheelFrontLeft/1
  WheelFrontRight Roll/1 -> WheelFrontRight/1
  WheelFrontRight Pitch/1 -> WheelFrontRight/2
  WheelRearLeft Roll/1 -> WheelRearLeft/1
  WheelRearLeft Pitch/1 -> WheelRearLeft/2
  WheelRearRight Roll/1 -> WheelRearRight/1
  WheelRearRight Ptich/1 -> WheelRearRight/2

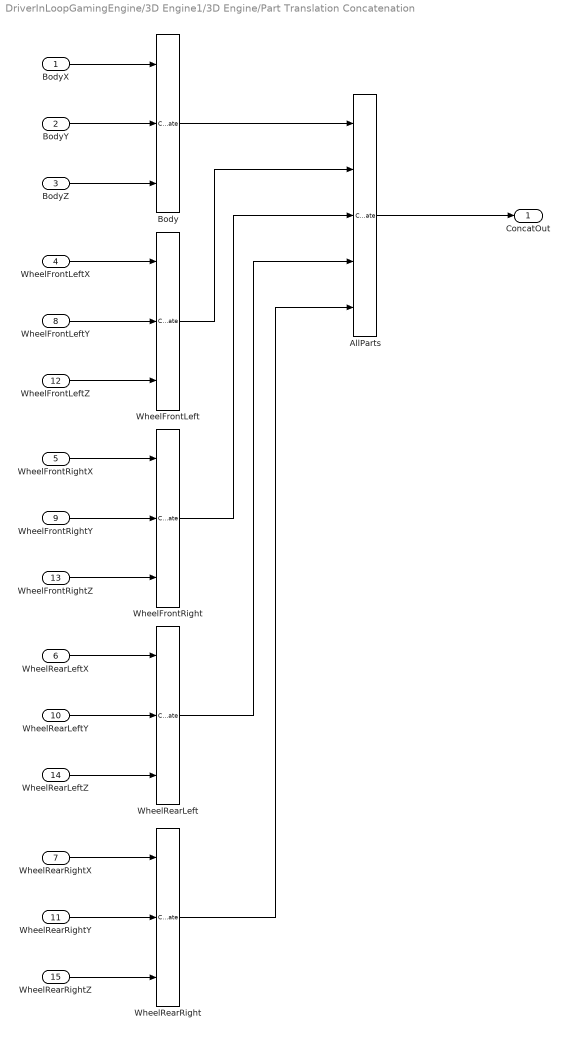
== system DriverInLoopGamingEngine/3D Engine1/3D Engine/Part Translation Concatenation ==
  BodyX : Inport
  BodyY : Inport  Port=2
  BodyZ : Inport  Port=3
  WheelFrontLeftX : Inport  Port=4
  WheelFrontRightX : Inport  Port=5
  WheelRearLeftX : Inport  Port=6
  WheelRearRightX : Inport  Port=7
  WheelFrontLeftY : Inport  Port=8
  WheelFrontRightY : Inport  Port=9
  WheelRearLeftY : Inport  Port=10
  WheelRearRightY : Inport  Port=11
  WheelFrontLeftZ : Inport  Port=12
  WheelFrontRightZ : Inport  Port=13
  WheelRearLeftZ : Inport  Port=14
  WheelRearRightZ : Inport  Port=15
  AllParts : Concatenate  NumInputs=5  Mode=Multidimensional array
  Body : Concatenate  NumInputs=3  Mode=Multidimensional array  ConcatenateDimension=2
  WheelFrontLeft : Concatenate  NumInputs=3  Mode=Multidimensional array  ConcatenateDimension=2
  WheelFrontRight : Concatenate  NumInputs=3  Mode=Multidimensional array  ConcatenateDimension=2
  WheelRearLeft : Concatenate  NumInputs=3  Mode=Multidimensional array  ConcatenateDimension=2
  WheelRearRight : Concatenate  NumInputs=3  Mode=Multidimensional array  ConcatenateDimension=2
  ConcatOut : Outport  VectorParamsAs1DForOutWhenUnconnected=off
  wires:
  BodyX/1 -> Body/1
  BodyZ/1 -> Body/3
  WheelFrontLeftX/1 -> WheelFrontLeft/1
  WheelFrontLeftZ/1 -> WheelFrontLeft/3
  WheelFrontLeftY/1 -> WheelFrontLeft/2
  BodyY/1 -> Body/2
  WheelFrontLeft/1 -> AllParts/2
  WheelRearRightX/1 -> WheelRearRight/1
  Body/1 -> AllParts/1
  WheelRearLeft/1 -> AllParts/4
  WheelFrontRight/1 -> AllParts/3
  WheelRearRightZ/1 -> WheelRearRight/3
  WheelFrontRightY/1 -> WheelFrontRight/2
  WheelFrontRightX/1 -> WheelFrontRight/1
  WheelRearRightY/1 -> WheelRearRight/2
  WheelRearLeftZ/1 -> WheelRearLeft/3
  AllParts/1 -> ConcatOut/1
  WheelRearLeftY/1 -> WheelRearLeft/2
  WheelRearRight/1 -> AllParts/5
  WheelRearLeftX/1 -> WheelRearLeft/1
  WheelFrontRightZ/1 -> WheelFrontRight/3

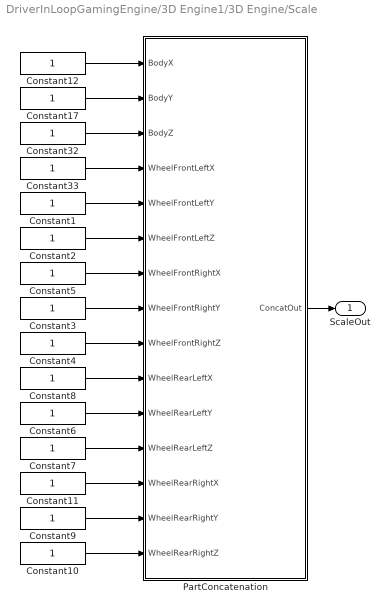
== system DriverInLoopGamingEngine/3D Engine1/3D Engine/Scale ==
  Constant{1..12,17,32..33} (15 alike) : Constant  OutDataTypeStr=single
  PartConcatenation : Subsystem
  ScaleOut : Outport  VectorParamsAs1DForOutWhenUnconnected=off
  wires:
  Constant10/1 -> PartConcatenation/15(WheelRearRightZ)
  Constant9/1 -> PartConcatenation/14(WheelRearRightY)
  Constant11/1 -> PartConcatenation/13(WheelRearRightX)
  Constant7/1 -> PartConcatenation/12(WheelRearLeftZ)
  Constant6/1 -> PartConcatenation/11(WheelRearLeftY)
  Constant8/1 -> PartConcatenation/10(WheelRearLeftX)
  Constant4/1 -> PartConcatenation/9(WheelFrontRightZ)
  Constant3/1 -> PartConcatenation/8(WheelFrontRightY)
  Constant5/1 -> PartConcatenation/7(WheelFrontRightX)
  Constant2/1 -> PartConcatenation/6(WheelFrontLeftZ)
  Constant1/1 -> PartConcatenation/5(WheelFrontLeftY)
  Constant33/1 -> PartConcatenation/4(WheelFrontLeftX)
  Constant32/1 -> PartConcatenation/3(BodyZ)
  Constant17/1 -> PartConcatenation/2(BodyY)
  Constant12/1 -> PartConcatenation/1(BodyX)
  PartConcatenation/1(ConcatOut) -> ScaleOut/1

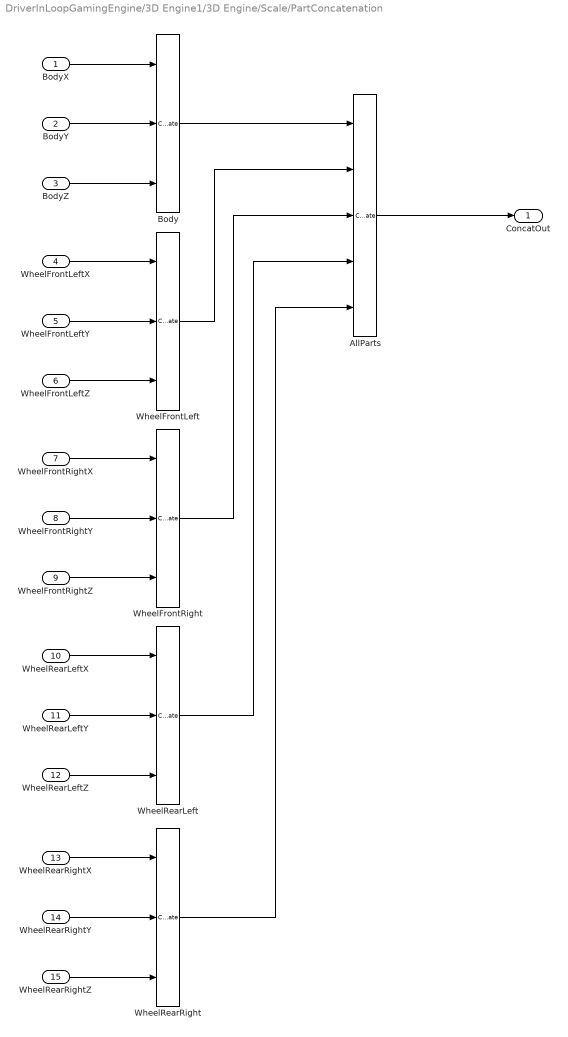
== system DriverInLoopGamingEngine/3D Engine1/3D Engine/Scale/PartConcatenation ==
  BodyX : Inport
  BodyY : Inport  Port=2
  BodyZ : Inport  Port=3
  WheelFrontLeftX : Inport  Port=4
  WheelFrontLeftY : Inport  Port=5
  WheelFrontLeftZ : Inport  Port=6
  WheelFrontRightX : Inport  Port=7
  WheelFrontRightY : Inport  Port=8
  WheelFrontRightZ : Inport  Port=9
  WheelRearLeftX : Inport  Port=10
  WheelRearLeftY : Inport  Port=11
  WheelRearLeftZ : Inport  Port=12
  WheelRearRightX : Inport  Port=13
  WheelRearRightY : Inport  Port=14
  WheelRearRightZ : Inport  Port=15
  AllParts : Concatenate  NumInputs=5  Mode=Multidimensional array
  Body : Concatenate  NumInputs=3  Mode=Multidimensional array  ConcatenateDimension=2
  WheelFrontLeft : Concatenate  NumInputs=3  Mode=Multidimensional array  ConcatenateDimension=2
  WheelFrontRight : Concatenate  NumInputs=3  Mode=Multidimensional array  ConcatenateDimension=2
  WheelRearLeft : Concatenate  NumInputs=3  Mode=Multidimensional array  ConcatenateDimension=2
  WheelRearRight : Concatenate  NumInputs=3  Mode=Multidimensional array  ConcatenateDimension=2
  ConcatOut : Outport  VectorParamsAs1DForOutWhenUnconnected=off
  wires:
  BodyX/1 -> Body/1
  BodyZ/1 -> Body/3
  WheelFrontLeftX/1 -> WheelFrontLeft/1
  WheelFrontLeftZ/1 -> WheelFrontLeft/3
  WheelFrontLeftY/1 -> WheelFrontLeft/2
  BodyY/1 -> Body/2
  WheelFrontLeft/1 -> AllParts/2
  WheelRearRightX/1 -> WheelRearRight/1
  Body/1 -> AllParts/1
  WheelRearLeft/1 -> AllParts/4
  WheelFrontRight/1 -> AllParts/3
  WheelRearRightZ/1 -> WheelRearRight/3
  WheelFrontRightY/1 -> WheelFrontRight/2
  WheelFrontRightX/1 -> WheelFrontRight/1
  WheelRearRightY/1 -> WheelRearRight/2
  WheelRearLeftZ/1 -> WheelRearLeft/3
  AllParts/1 -> ConcatOut/1
  WheelRearLeftY/1 -> WheelRearLeft/2
  WheelRearRight/1 -> AllParts/5
  WheelRearLeftX/1 -> WheelRearLeft/1
  WheelFrontRightZ/1 -> WheelFrontRight/3
